simulink model "mpu6050"  (R2017b)
settings: Solver=FixedStepDiscrete  StartTime=0.0  StopTime=0.5  FixedStep=0.01  RelTol=1e-3
undefined symbols (not defined in the file): DiscIntNeverNeededParam, KiRollAttitude, KpRollAttitude, mpu6050
libraries: simulink x6, GPIO_Lib x3, TIMERS_Lib x2, STM32_Config_Lib x1
(part 2 of 2)

== system mpu6050/Subsystem2/Subsystem2 ==
  In1 : Inport
  Constant3 : Constant  Value=1500  OutDataTypeStr=single
  Constant4 : Constant  Value=500  OutDataTypeStr=single
  Dead Zone : DeadZone  LowerValue=-70  UpperValue=70  SaturateOnIntegerOverflow=on
  Divide1 : Product  Inputs=*/
  Saturation4 : Saturate  UpperLimit=2000  LowerLimit=1000
  Sum1 : Sum  Inputs=|+-
  Out1 : Outport
  wires:
  Sum1/1 -> Dead Zone/1
  In1/1 -> Saturation4/1
  Constant4/1 -> Divide1/2
  Saturation4/1 -> Sum1/1
  Constant3/1 -> Sum1/2
  Dead Zone/1 -> Divide1/1
  Divide1/1 -> Out1/1

== system mpu6050/Subsystem2/Subsystem3 ==
  In1 : Inport
  Constant3 : Constant  Value=1500  OutDataTypeStr=single
  Constant4 : Constant  Value=500  OutDataTypeStr=single
  Dead Zone : DeadZone  LowerValue=-70  UpperValue=70  SaturateOnIntegerOverflow=on
  Divide1 : Product  Inputs=*/
  Saturation4 : Saturate  UpperLimit=2000  LowerLimit=1000
  Sum1 : Sum  Inputs=|+-
  Out1 : Outport
  wires:
  Sum1/1 -> Dead Zone/1
  In1/1 -> Saturation4/1
  Constant4/1 -> Divide1/2
  Saturation4/1 -> Sum1/1
  Constant3/1 -> Sum1/2
  Dead Zone/1 -> Divide1/1
  Divide1/1 -> Out1/1

== system mpu6050/Subsystem2/Subsystem4 ==
  In1 : Inport
  Constant3 : Constant  Value=1000  OutDataTypeStr=single
  Saturation4 : Saturate  UpperLimit=2000  LowerLimit=1000
  Sum1 : Sum  Inputs=|+-
  Out1 : Outport
  wires:
  Constant3/1 -> Sum1/2
  Saturation4/1 -> Sum1/1
  In1/1 -> Saturation4/1
  Sum1/1 -> Out1/1

== system mpu6050/Yaw1/If Action Subsystem ==
  In1 : Inport
  Action Port : ActionPort  ActionType=then
  Out1 : Outport
  wires:
  In1/1 -> Out1/1

== system mpu6050/Yaw1/If Action Subsystem1 ==
  In1 : Inport
  Action Port : ActionPort  ActionType=else
  Out1 : Outport
  wires:
  In1/1 -> Out1/1

== system mpu6050/Yaw1/限幅到+-180 ==
  In1 : Inport  OutDataTypeStr=single
  Add : Sum
  Add1 : Sum
  Constant : Constant  Value=-360  OutDataTypeStr=single
  Constant1 : Constant  Value=360  OutDataTypeStr=single
  If : If  IfExpression=u1 > 180  ElseIfExpressions=u1 < -180
  If Action Subsystem : Subsystem  TreatAsAtomicUnit=on
  If Action Subsystem1 : Subsystem  TreatAsAtomicUnit=on
  If Action Subsystem2 : Subsystem  TreatAsAtomicUnit=on
  Merge : Merge  Inputs=3
  Out1 : Outport
  wires:
  In1/1 -> Add1/2, If Action Subsystem2/1(In1), Add/2, If/1
  If/1 -> If Action Subsystem/Action
  If/2 -> If Action Subsystem1/Action
  If/3 -> If Action Subsystem2/Action
  If Action Subsystem/1(Out1) -> Merge/1
  Constant/1 -> Add/1
  Add/1 -> If Action Subsystem/1(In1)
  If Action Subsystem1/1(Out1) -> Merge/2
  Constant1/1 -> Add1/1
  If Action Subsystem2/1(Out1) -> Merge/3
  Add1/1 -> If Action Subsystem1/1(In1)
  Merge/1 -> Out1/1

== system mpu6050/Yaw1/限幅到+-180，， ==
  In1 : Inport  OutDataTypeStr=single
  Add : Sum
  Add1 : Sum
  Constant : Constant  Value=-360  OutDataTypeStr=single
  Constant1 : Constant  Value=360  OutDataTypeStr=single
  If : If  IfExpression=u1 > 180  ElseIfExpressions=u1 < -180
  If Action Subsystem : Subsystem  TreatAsAtomicUnit=on
  If Action Subsystem1 : Subsystem  TreatAsAtomicUnit=on
  If Action Subsystem2 : Subsystem  TreatAsAtomicUnit=on
  Merge : Merge  Inputs=3
  Out1 : Outport
  wires:
  In1/1 -> Add1/2, If Action Subsystem2/1(In1), Add/2, If/1
  If/1 -> If Action Subsystem/Action
  If/2 -> If Action Subsystem1/Action
  If/3 -> If Action Subsystem2/Action
  If Action Subsystem/1(Out1) -> Merge/1
  Constant/1 -> Add/1
  Add/1 -> If Action Subsystem/1(In1)
  If Action Subsystem1/1(Out1) -> Merge/2
  Constant1/1 -> Add1/1
  If Action Subsystem2/1(Out1) -> Merge/3
  Add1/1 -> If Action Subsystem1/1(In1)
  Merge/1 -> Out1/1

== system mpu6050/judgeLock2/If Action Subsystem ==
  In1 : Inport
  Action Port : ActionPort  ActionType=then
  Out1 : Outport
  wires:
  In1/1 -> Out1/1

== system mpu6050/judgeLock2/If Action Subsystem1 ==
  In1 : Inport
  Action Port : ActionPort  ActionType=else
  Out1 : Outport
  wires:
  In1/1 -> Out1/1

== system mpu6050/限幅到+-180，/If Action Subsystem ==
  In1 : Inport
  Action Port : ActionPort  ActionType=then
  Out1 : Outport
  wires:
  In1/1 -> Out1/1

== system mpu6050/限幅到+-180，/If Action Subsystem1 ==
  In1 : Inport
  Action Port : ActionPort  ActionType=elseif
  Out1 : Outport
  wires:
  In1/1 -> Out1/1

== system mpu6050/限幅到+-180，/If Action Subsystem2 ==
  In1 : Inport
  Action Port : ActionPort  ActionType=else
  Out1 : Outport
  wires:
  In1/1 -> Out1/1

== system mpu6050/PWM1/Subsystem/If Action Subsystem ==
  In1 : Inport
  Action Port : ActionPort  ActionType=then
  Out1 : Outport
  wires:
  In1/1 -> Out1/1

== system mpu6050/PWM1/Subsystem/If Action Subsystem1 ==
  In1 : Inport
  Action Port : ActionPort  ActionType=else
  Out1 : Outport
  wires:
  In1/1 -> Out1/1

== system mpu6050/State Estimation and Complimentary Mixing1/Complimentary Filter/Filter IC fixer ==
  FilterStart : Inport
  Normal Output : Inport  Port=2
  Constant : Constant
  IC : InitialCondition  Value=0
  Switch : Switch  Criteria=u2 ~= 0
  Out1 : Outport
  wires:
  Switch/1 -> Out1/1
  FilterStart/1 -> Switch/3
  IC/1 -> Switch/2
  Constant/1 -> IC/1
  Normal Output/1 -> Switch/1

== system mpu6050/State Estimation and Complimentary Mixing1/Complimentary Filter/Filter IC fixer1 ==
  FilterStart : Inport
  Normal Output : Inport  Port=2
  Constant : Constant
  IC : InitialCondition  Value=0
  Switch : Switch  Criteria=u2 ~= 0
  Out1 : Outport
  wires:
  Switch/1 -> Out1/1
  FilterStart/1 -> Switch/3
  IC/1 -> Switch/2
  Constant/1 -> IC/1
  Normal Output/1 -> Switch/1

== system mpu6050/State Estimation and Complimentary Mixing1/Complimentary Filter/Filter IC fixer2 ==
  FilterStart : Inport
  Normal Output : Inport  Port=2
  Constant : Constant
  IC : InitialCondition  Value=0
  Switch : Switch  Criteria=u2 ~= 0
  Out1 : Outport
  wires:
  Switch/1 -> Out1/1
  FilterStart/1 -> Switch/3
  IC/1 -> Switch/2
  Constant/1 -> IC/1
  Normal Output/1 -> Switch/1

== system mpu6050/State Estimation and Complimentary Mixing1/Subsystem1/Magnitude ==
  x_acc : Inport
  y_acc : Inport  Port=2
  z_acc : Inport  Port=3
  Demux1 : Demux  Outputs=3
  Math Function : Math  Operator=square  SaturateOnIntegerOverflow=on
  Mux : Mux  Inputs=3
  Sqrt : Sqrt  SaturateOnIntegerOverflow=on
  Sum : Sum  Inputs=+++
  |g| : Outport
  wires:
  Sqrt/1 -> |g|/1  "mag_acc"
  Sum/1 -> Sqrt/1
  Demux1/3 -> Sum/3
  Mux/1 -> Math Function/1
  Math Function/1 -> Demux1/1
  Demux1/1 -> Sum/1
  Demux1/2 -> Sum/2
  y_acc/1 -> Mux/2
  x_acc/1 -> Mux/1
  z_acc/1 -> Mux/3

== system mpu6050/Yaw1/限幅到+-180/If Action Subsystem ==
  In1 : Inport
  Action Port : ActionPort  ActionType=then
  Out1 : Outport
  wires:
  In1/1 -> Out1/1

== system mpu6050/Yaw1/限幅到+-180/If Action Subsystem1 ==
  In1 : Inport
  Action Port : ActionPort  ActionType=elseif
  Out1 : Outport
  wires:
  In1/1 -> Out1/1

== system mpu6050/Yaw1/限幅到+-180/If Action Subsystem2 ==
  In1 : Inport
  Action Port : ActionPort  ActionType=else
  Out1 : Outport
  wires:
  In1/1 -> Out1/1

== system mpu6050/Yaw1/限幅到+-180，，/If Action Subsystem ==
  In1 : Inport
  Action Port : ActionPort  ActionType=then
  Out1 : Outport
  wires:
  In1/1 -> Out1/1

== system mpu6050/Yaw1/限幅到+-180，，/If Action Subsystem1 ==
  In1 : Inport
  Action Port : ActionPort  ActionType=elseif
  Out1 : Outport
  wires:
  In1/1 -> Out1/1

== system mpu6050/Yaw1/限幅到+-180，，/If Action Subsystem2 ==
  In1 : Inport
  Action Port : ActionPort  ActionType=else
  Out1 : Outport
  wires:
  In1/1 -> Out1/1

== stateflow chart mpu6050/Attitude1/pitchAngle ==
  (default) -> (junction 2) : {kp=ctrl_2.PID[PIDPITCH].kp;ki=ctrl_2.PID[PIDPITCH].ki;kd=ctrl_2.PID[PIDPITCH].kd}
  data: kp output single; ki output single; kd output single

== stateflow chart mpu6050/Chart3 ==
  note: 
  note: 第一步设置动作语言为C语言
  (default) -> (junction 17)
  (junction 17) -> (junction 19) : {IMUSO3Thread(gyroData,accData,ouler);
      | }
  data: gyroData input single size=3*1 =0; accData input single size=3*1 =0; ouler output single size=3*1

== stateflow chart mpu6050/Attitude1/rollAngle ==
  (default) -> (junction 2) : {kp=ctrl_2.PID[PIDROLL].kp;ki=ctrl_2.PID[PIDROLL].ki;kd=ctrl_2.PID[PIDROLL].kd}
  data: kp output single; ki output single; kd output single

== stateflow chart mpu6050/Attitude1/rollRate ==
  (default) -> (junction 2) : {kp=ctrl_1.PID[PIDROLL].kp;ki=ctrl_1.PID[PIDROLL].ki;kd=ctrl_1.PID[PIDROLL].kd}
  data: kp output single; ki output single; kd output single

== stateflow chart mpu6050/Attitude1/pitchRate ==
  (default) -> (junction 2) : {kp=ctrl_1.PID[PIDPITCH].kp;ki=ctrl_1.PID[PIDPITCH].ki;kd=ctrl_1.PID[PIDPITCH].kd}
  data: kp output single; ki output single; kd output single

== stateflow chart mpu6050/Chart2 ==
  (default) -> (junction 4)
  (junction 4) -> (junction 6) : {ANO_DT_Data_Receive_Prepare(data);}
  data: data input uint8

== stateflow chart mpu6050/Yaw1/Chart1 ==
  (default) -> (junction 4)
  (junction 4) -> (junction 6) : {ANO_DT_Send_Status(roll, pitch, yaw,0,0,0);}
  data: roll input single size=1; pitch input single size=1; yaw input single size=1

== stateflow chart mpu6050/Chart4 ==
  (default) -> (junction 4)
  (junction 4) -> (junction 6) : {ANO_DT_Send_Senser(accData[0],accData[1],accData[2],gyroData[0],gyroData[1],gyroData[2],0,0,0,0);}
  data: gyroData input; accData input

== stateflow chart mpu6050/controller ==
  (default) -> (junction 8)
  (junction 8) -> (junction 10) : {RC_DATA.ROLL=rollInput;RC_DATA.PITCH=pitchInput;
      | RC_DATA.YAW=yawInput;Thro=throInput;
      | controller();
      | rollOutSim=RollOut;pitchOutSim=PitchOut;yawOutSim=YawOut;}
  data: rollOutSim output single; pitchOutSim output single; yawInput input single; pitchInput input single; rollInput input single; throInput input single; yawOutSim output single

== stateflow chart mpu6050/sensor ==
  (default) -> (junction 10)
  (junction 10) -> (junction 12) : {imu.gyro[ROLL1]=pInput;imu.gyro[PITCH2]=qInput;imu.gyro[YAW3]=rInput;
      | imu.roll=rollInput;imu.pitch=pitchInput;imu.yaw=yawInput;}
  data: yawInput input single; pitchInput input single; rollInput input single; pInput input single; qInput input single; rInput input single

== stateflow chart mpu6050/Chart5 ==
  note: 
  note: 第一步设置动作语言为C语言
  state checkLock [function]
    (default) -> (junction 62)
    (junction 62) -> (junction 63) [order 1] : [FlyOk==0&&(rcDataTmp[2]<1080)&&(rcDataTmp[3]>1990)]{OpenLock=OpenLock+1}
    (junction 63) -> (junction 65) : [OpenLock>200]{FlyOk=1;OpenLock=200;}
    (junction 62) -> (junction 64) [order 2] : [FlyOk==1&&(rcDataTmp[2]<1080)&&(rcDataTmp[3]<1010)]{OpenLock=OpenLock-1}
    (junction 64) -> (junction 66) : [OpenLock<0]{OpenLock=0;FlyOk=0;}
  (default) -> (junction 72)
  (junction 72) -> (junction 74) : {receiveData(rcDataTmp);
      | checkLock();ANO_DT_Data_Exchange();}
  data: rcDataTmp output uint16 size=4*1 =0; OpenLock local int16 size=1 =0; FlyOk output int8 size=1 =0

== stateflow chart mpu6050/PWM1/Chart1 ==
  (default) -> (junction 4)
  (junction 4) -> (junction 6) : {ANO_DT_Send_MotoPWM(m_1,m_2,m_3,m_4,0,0,0,0);}
  data: m_1 input; m_2 input; m_3 input; m_4 input

== matlab function mpu6050/pwm_out2 ==
  data: Roll input; M1 output; Pitch input; Yaw input; Thrust input; M2 output; M3 output; M4 output; thrLow input
function [M1, M2, M3, M4] = motor_mixer(Roll, Pitch, Yaw, Thrust,thrLow)

% idle_PWM = uint16(1000);

% Quad X/ 2000 * Thrust
M1 = ((Roll - Pitch - Yaw)* thrLow  + 0.5*Thrust) ;
M2 = ((-Roll - Pitch + Yaw)* thrLow  + 0.5*Thrust) ;
M3 = ((-Roll + Pitch - Yaw)* thrLow + 0.5*Thrust) ;
M4 = ((Roll + Pitch + Yaw)* thrLow + 0.5*Thrust);
% M5 = 1000;
% M6 = 1000;
% M7 = 1000;
% M8 = 1000;

% Quad +
% M1 = ((Pitch - Yaw) * Thrust / 2 + Thrust) * 1000 + idle_PWM;
% M2 = ((-Roll + Yaw) * Thrust / 2 + Thrust) * 1000 + idle_PWM;
% M3 = ((-Pitch - Yaw) * Thrust / 2 + Thrust) * 1000 + idle_PWM;
% M4 = ((Roll + Yaw) * Thrust / 2 + Thrust) * 1000 + idle_PWM;
% M5 = 1000;
% M6 = 1000;
% M7 = 1000;
% M8 = 1000;

% Hex X
% M1 = ((Pitch + Roll / 2 - Yaw) * Thrust / 2 + Thrust) * 1000 + idle_PWM;
% M2 = ((Pitch - Roll / 2 + Yaw) * Thrust / 2 + Thrust) * 1000 + idle_PWM;
% M3 = ((-Roll - Yaw) * Thrust / 2 + Thrust) * 1000 + idle_PWM;
% M4 = ((-Pitch - Roll / 2 + Yaw) * Thrust / 2 + Thrust) * 1000 + idle_PWM;
% M5 = ((-Pitch + Roll / 2 - Yaw) * Thrust / 2 + Thrust) * 1000 + idle_PWM;
% M6 = ((Roll + Yaw) * Thrust / 2 + Thrust) * 1000 + idle_PWM;
% M7 = 1000;
% M8 = 1000;

% Hex X (From Adam)
% M1 = uint16(single(((-Roll - Yaw) * Thrust / 3 + Thrust) * single(1000))) + idle_PWM;
% M2 = uint16(single(((Roll + Yaw) * Thrust / 3 + Thrust) * single(1000))) + idle_PWM;
% M3 = uint16(single(((Pitch + (Roll / 2) - Yaw) * Thrust / 3 + Thrust) * single(1000))) + idle_PWM;
% M4 = uint16(single(((-Pitch - (Roll / 2) + Yaw) * Thrust / 3 + Thrust) * single(1000))) + idle_PWM;
% M5 = uint16(single(((Pitch - (Roll / 2) + Yaw) * Thrust / 3 + Thrust) * single(1000))) + idle_PWM;
% M6 = uint16(single(((-Pitch + (Roll / 2) - Yaw) * Thrust / 3 + Thrust) * single(1000))) + idle_PWM;

% Hex X (Version 2)
% Roll/Yaw
% M1 = ((-Roll - Yaw) * Thrust / 2 + Thrust) * 1000 + idle_PWM;
% M2 = ((Roll + Yaw) * Thrust / 2 + Thrust) * 1000 + idle_PWM;
% % + Pitch/Roll
% M6 = ((Pitch + Roll / 2 - Yaw) * Thrust / 2 + Thrust) * 1000 + idle_PWM;
% M4 = ((Pitch - Roll / 2 + Yaw) * Thrust / 2 + Thrust) * 1000 + idle_PWM;
% % - Pitch/Roll
% M5 = ((-Pitch - Roll / 2 + Yaw) * Thrust / 2 + Thrust) * 1000 + idle_PWM;
% M3 = ((-Pitch + Roll / 2 - Yaw) * Thrust / 2 + Thrust) * 1000 + idle_PWM;

== stateflow chart mpu6050/Chart1 ==
  (default) -> (junction 4)
  (junction 4) -> (junction 6) : {ANO_DT_Send_Status(roll, pitch, yaw,0,0,0);}
  data: roll input single size=1; pitch input single size=1; yaw input single size=1

== stateflow chart mpu6050/Chart6 ==
  state offset=calOffset(gyro_x,gyro_y,gyro_z,acc_x,acc_y,acc_z) [function]
  (default) -> (junction 16) : /* calOffset */
  (junction 16) -> (junction 17) [order 1] : [i<100]
  (junction 16) -> (junction 18) [order 2] : [i>=100]
  (junction 17) -> (junction 19) : {i++;offset=calOffset(gx,gy,gz,ax,ay,az);}
  (junction 19) -> (junction 18)
  (junction 18) -> (junction 20)
  data: gyro_x function_input int32; gyro_y function_input int32; gyro_z function_input int32; acc_x function_input int32; acc_y function_input int32; acc_z function_input int32; offset function_output single; ax input int32; ay input int32; az input int32; gx input int32; gy input int32; gz input int32; i local int16 size=1 =0; offset output int32 size=6*1

== stateflow chart mpu6050/Chart7 ==
  note: 
  note: 第一步设置动作语言为C语言
  note: ANO_DT_Send_Senser(accData[0],accData[1],accData[2],gyroData[0],gyroData[1],gyroData[2],0,0,0,0);
  (default) -> (junction 17)
  (junction 17) -> (junction 19) : {MPU6050ReadGyro(gyroData);
      | MPU6050ReadAcc(accData);
      | }
  data: gyroData output int16 size=3*1 =0; accData output int16 size=3*1 =0

== stateflow chart mpu6050/Chart8 ==
  state pwmInit [function]
  state BTInit [function]
  (default) -> (junction 16) : /* init */
  (junction 16) -> (junction 17) [order 1] : [i<1]
  (junction 16) -> (junction 18) [order 2] : [i>=1]
  (junction 17) -> (junction 19) : {pwmInit();BTInit();I2C_InitGPIO();MPU6050_Init();NRF24L01_SPI_Init();ParamSetDefault();i++;}
  (junction 19) -> (junction 18)
  (junction 18) -> (junction 20)
  data: i local int8 size=1 =0
